simulink model "Essai_CPU_couleur"  (R2021a)
settings: Solver=FixedStepAuto  StartTime=0.0  StopTime=inf  RelTol=1e-3  EnableMultiTasking=on
libraries: arduinolib x6, dspstat3 x2, simulink x1
settings Model: SILPILModeSetting=veronly  ExtModeTrigDuration=2  Creator=Etudiant  LastModifiedBy=ethan
settings SolverCC: AlgebraicLoopSolver=TrustRegion
settings OptimizationCC: EnhancedBackFolding=on  PassReuseOutputArgsAs=Individual arguments  ZeroExternalMemoryAtStartup=off  ZeroInternalMemoryAtStartup=off  MaxStackSize=64  OptimizeBlockOrder=speed  DifferentSizesBufferReuse=on  OptimizationCustomize=off  EfficientTunableParamExpr=on
settings DebuggingCC: ParameterPrecisionLossMsg=none  ParameterTunabilityLossMsg=error  SFMachineParentedDataDiag=warning
settings HardwareCC: ProdBitPerInt=16  ProdBitPerPointer=16  ProdBitPerSizeT=16  ProdBitPerPtrDiffT=16  ProdLargestAtomicFloat=None  ProdWordSize=8  ProdHWDeviceType=Atmel->AVR
settings SFSimCC: MATLABDynamicMemAlloc=off
settings RTWCC: SystemTargetFile=ert.tlc  HardwareBoard=Arduino Mega 2560  TemplateMakefile=ert_default_tmf  CustomSource=enc_eml_src.c  Toolchain=Arduino AVR  BuildConfiguration=Faster Runs  IncludeHyperlinkInReport=on
settings CodeAppCC: ForceParamTrailComments=on  GenerateComments=off  IgnoreCustomStorageClasses=off  OperatorAnnotations=on  SimulinkDataObjDesc=on  SFDataObjDesc=on  InsertBlockDesc=on
settings ERTTargetCC: SupportContinuousTime=on  SupportVariableSizeSignals=on  ExtModeStaticAllocSize=2048

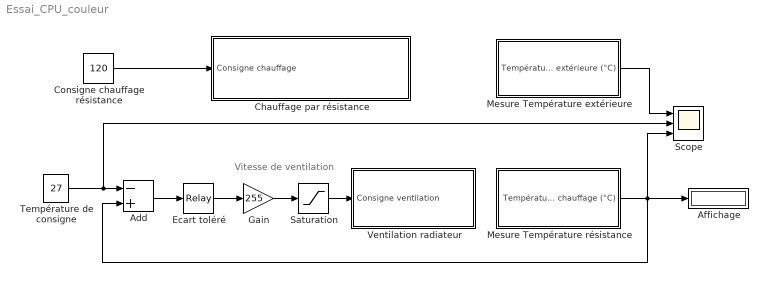
== system Essai_CPU_couleur ==
  note: Vitesse de ventilation
  Add : Sum  Inputs=-+
  Affichage : Display
  Chauffage par résistance : Subsystem
  "Consigne chauffage résistance " : Constant  Value=120  SampleTime=-1
  Ecart toléré : Relay  OnSwitchValue=2  OffSwitchValue=0
  Gain : Gain  Gain=255
  Mesure Température extérieure : Subsystem
  Mesure Température résistance : Subsystem
  Saturation : Saturate  UpperLimit=255  LowerLimit=0
  Scope : Scope  NumInputPorts=3
  Température de consigne : Constant  Value=27  SampleTime=0.01
  Ventilation radiateur : Subsystem
  wires:
  Saturation/1 -> Ventilation radiateur/1(Consigne ventilation)
  Add/1 -> Ecart toléré/1
  Ecart toléré/1 -> Gain/1
  Gain/1 -> Saturation/1
  "Consigne chauffage résistance "/1 -> Chauffage par résistance/1(Consigne chauffage)
  Température de consigne/1 -> Scope/2, Add/1
  Mesure Température résistance/1(Température chauffage (°C)) -> Affichage/1, Add/2, Scope/3
  Mesure Température extérieure/1(Température extérieure (°C)) -> Scope/1

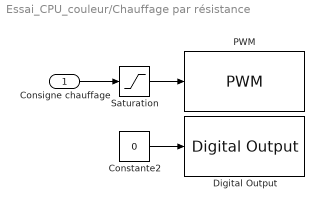
== system Essai_CPU_couleur/Chauffage par résistance ==
  Consigne chauffage : Inport
  Constante2 : Constant  Value=0  SampleTime=-1
  Digital Output : arduinolib/Digital Output  pinNumber=9  blockPlatform=arduino
  PWM : arduinolib/PWM  pinNumber=6  EnableInputFrequency=off  InitialFrequency=2000  InitialDutyCycle=0  NotificationType=None  blockPlatform=arduino
  Saturation : Saturate  UpperLimit=255  LowerLimit=0
  wires:
  Constante2/1 -> Digital Output/1
  Saturation/1 -> PWM/1
  Consigne chauffage/1 -> Saturation/1

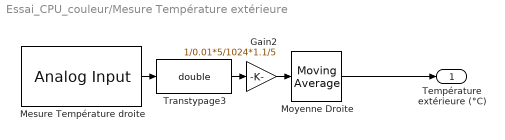
== system Essai_CPU_couleur/Mesure Température extérieure ==
  Gain2 : Gain  Gain=1/0.01*5/1024*1.1/5
  Mesure Température droite : arduinolib/Analog Input  pinNumber=2  ReadResultsOnly=off  ConversionTriggerSource=Software  ExternalTriggerType=uint32(0)  OutputDataType=uint16  EnableConversionCompleteNotify=off  EnableOuputStatus=off  SampleTime=-1  blockPlatform=arduino
  Moyenne Droite : dspstat3/Moving Average  Method=Sliding window  ForgettingFactorPort=off  SpecifyWindowLength=on  WindowLength=5  ForgettingFactor=0.9  SimulateUsing=Code generation
  Transtypage3 : DataTypeConversion  OutDataTypeStr=double
  Température extérieure (°C) : Outport
  wires:
  Gain2/1 -> Moyenne Droite/1
  Moyenne Droite/1 -> Température extérieure (°C)/1
  Mesure Température droite/1 -> Transtypage3/1
  Transtypage3/1 -> Gain2/1

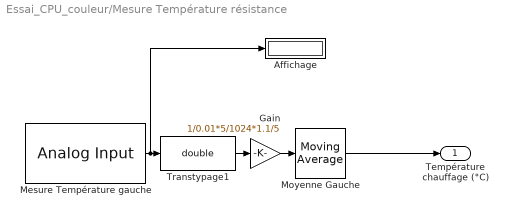
== system Essai_CPU_couleur/Mesure Température résistance ==
  Affichage : Display
  Gain : Gain  Gain=1/0.01*5/1024*1.1/5
  Mesure Température gauche : arduinolib/Analog Input  pinNumber=0  ReadResultsOnly=off  ConversionTriggerSource=Software  ExternalTriggerType=uint32(0)  OutputDataType=uint16  EnableConversionCompleteNotify=off  EnableOuputStatus=off  SampleTime=-1  blockPlatform=arduino
  Moyenne Gauche : dspstat3/Moving Average  Method=Sliding window  ForgettingFactorPort=off  SpecifyWindowLength=on  WindowLength=5  ForgettingFactor=0.9  SimulateUsing=Code generation
  Transtypage1 : DataTypeConversion  OutDataTypeStr=double
  Température chauffage (°C) : Outport
  wires:
  Gain/1 -> Moyenne Gauche/1
  Mesure Température gauche/1 -> Affichage/1, Transtypage1/1
  Transtypage1/1 -> Gain/1
  Moyenne Gauche/1 -> Température chauffage (°C)/1

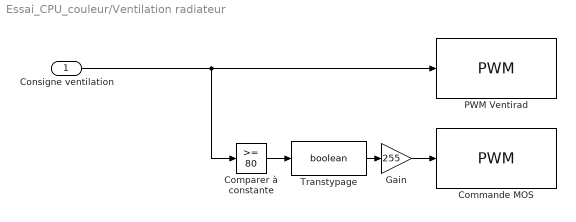
== system Essai_CPU_couleur/Ventilation radiateur ==
  Consigne ventilation : Inport
  Commande MOS : arduinolib/PWM  pinNumber=8  EnableInputFrequency=off  InitialFrequency=2000  InitialDutyCycle=0  NotificationType=None  blockPlatform=arduino
  Comparer à constante : simulink/Logic and Bit Operations/Compare To Constant  relop=>=  const=80  OutDataTypeStr=boolean
  Gain : Gain  Gain=255
  PWM Ventirad : arduinolib/PWM  pinNumber=12  EnableInputFrequency=off  InitialFrequency=2000  InitialDutyCycle=0  NotificationType=None  blockPlatform=arduino
  Transtypage : DataTypeConversion  OutDataTypeStr=boolean
  wires:
  Consigne ventilation/1 -> Comparer à constante/1, PWM Ventirad/1
  Transtypage/1 -> Gain/1
  Gain/1 -> Commande MOS/1
  Comparer à constante/1 -> Transtypage/1
